simulink model "generator_model_2023"  (R2023a)
settings: Solver=ode15s  StartTime=0.0  StopTime=0.2  FixedStep=1e-6  MaxStep=1e-5  RelTol=1e-5  EnableMultiTasking=on
InitFcn:
  | Rs=0.42;
  | Ls=0.96e-3;
  | C_phi=92.1952e-3;
  | poles=8;
  | Rload=15;
model workspace (MAT data in the model file):
  D = Simulink.Parameter
  D.Value = 0
  D.DataType = 'double'
  D.Complexity = 'real'
  D.Dimensions = [1 1]
  Power_previous = Simulink.Parameter
  Power_previous.Value = 0
  Power_previous.DataType = 'auto'
  Power_previous.Complexity = 'real'
  Power_previous.Dimensions = [1 1]
  R_eq = Simulink.Parameter
  R_eq.Value = 100
  R_eq.DataType = 'double'
  R_eq.Complexity = 'real'
  R_eq.Dimensions = [1 1]
  direction = Simulink.Parameter
  direction.Value = 0
  direction.DataType = 'auto'
  direction.Complexity = 'real'
  direction.Dimensions = [1 1]
libraries: spsDiodeLib x6, spsSeriesRLCBranchLib x6, spsControlledVoltageSourceLib x3, ee_lib x2, spsVoltageMeasurementLib x2, spsCurrentMeasurementLib x1, spsGroundLib x1, spsParallelRLCBranchLib x1, sps_lib x1
settings Model: Creator=jwjansen  LastModifiedBy=maarten
settings SolverCC: AlgebraicLoopSolver=TrustRegion
settings DataIOCC: LimitDataPoints=on  SaveFormat=Array  ReturnWorkspaceOutputs=off
settings OptimizationCC: ExpressionDepthLimit=2147483647  LifeSpan=inf
settings DebuggingCC: UnderspecifiedInitializationDetection=Classic  MergeDetectMultiDrivingBlocksExec=none  SolverPrmCheckMsg=warning  FcnCallInpInsideContextMsg=warning  StateNameClashWarn=warning  SFUnexpectedBacktrackingDiag=warning  SFNoUnconditionalDefaultTransitionDiag=warning  SFExecutionAtInitializationDiag=none  ArithmeticOperatorsInVariantConditions=warning
settings HardwareCC: ProdBitPerPointer=32  ProdBitPerSizeT=32  ProdBitPerPtrDiffT=32  ProdLargestAtomicFloat=None  ProdIntDivRoundTo=Undefined  ProdEndianess=Unspecified  ProdWordSize=32  ProdHWDeviceType=32-bit Generic
settings ModelReferenceCC: EnableRefExpFcnMdlSchedulingChecks=on  PropagateSignalLabelsOutOfModel=off
settings SFSimCC: SimUseLocalCustomCode=off  SimParseCustomCode=off  CustomCodeUndefinedFunction=UseInterfaceOnly
settings RTWCC: RTWUseLocalCustomCode=off
settings CodeAppCC: StateflowObjectComments=on
settings GRTTargetCC: TargetLangStandard=C89/C90 (ANSI)  CombineOutputUpdateFcns=off  GRTInterface=on
settings ConfigComp: CovMetricSettings=dw  CovSaveCumulativeToWorkspaceVar=on  CovSaveSingleToWorkspaceVar=on  CovExternalEMLEnable=off
settings SimscapeCC: SimscapeNormalizeSystem=off

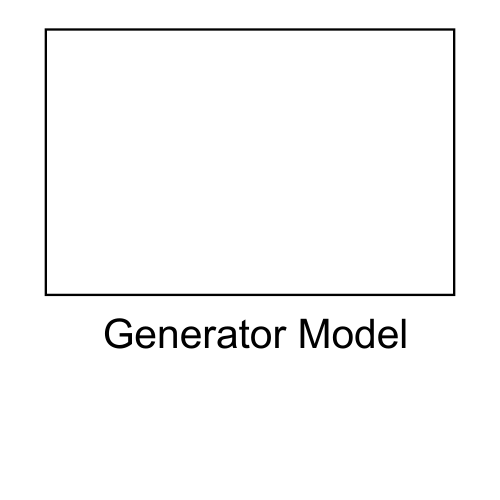
[thumbnail: Simulink's stored preview of the top-level diagram]
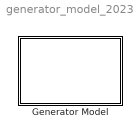
== system generator_model_2023 ==
  " Generator Model " : Subsystem

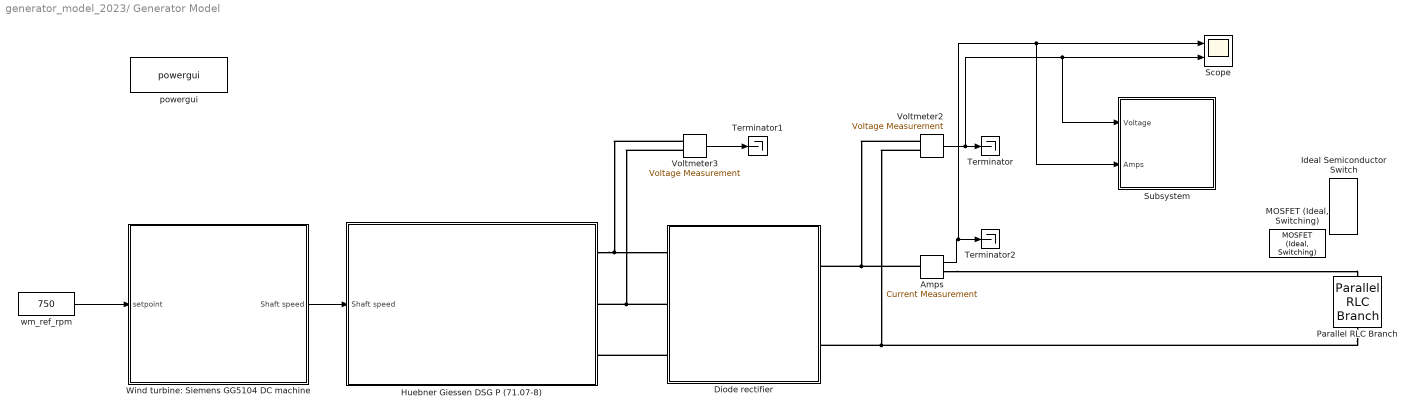
== system generator_model_2023/ Generator Model  ==
  Amps : spsCurrentMeasurementLib/Current Measurement  PhasorSimulation=off  OutputType=Complex  PSBequivalent=0
  Diode rectifier : Subsystem
  "Huebner Giessen DSG P (71.07-8) " : Subsystem
  Ideal Semiconductor Switch : ee_lib/Semiconductors & Converters/Ideal Semiconductor Switch  port_option=ee.enum.controlport.ps  Ron=0.001 Ohm  Goff=1e-6 1/Ohm  Vth=0.5 V  diode_param=ee.enum.converters.protectiondiode.none  diode_Vf=0.8 V  diode_Ron=0.001 Ohm  diode_Goff=1e-5 1/Ohm  diode_C=50e-9 F  diode_iRM=-235 A  diode_iF=300 A  diode_idot=-50 A/us  diode_trr_param=ee.enum.converters.diodetrr.trr_factor  diode_trr_factor=3  diode_trr=15 us  diode_Qrr=1500 s*uA
  "MOSFET (Ideal, Switching)" : ee_lib/Semiconductors & Converters/MOSFET (Ideal, Switching)  port_option=ee.enum.controlport.ps  Rds=0.01 Ohm  Goff=1e-6 1/Ohm  Vth=2 V  diode_param=ee.enum.converters.protectiondiode.none  diode_Vf=0.8 V  diode_Ron=0.001 Ohm  diode_Goff=1e-5 1/Ohm  diode_C=50e-9 F  diode_iRM=-235 A  diode_iF=300 A  diode_idot=-50 A/us  diode_trr_param=ee.enum.converters.diodeReverseParam.trr_factor  diode_trr_factor=3  diode_trr=15 us  diode_Qrr=1500 s*uA  ids_specify=off  ids_priority=None  ids=0 A  ids_nominal_specify=off  ids_nominal_unit=A  ids_nominal_value=1  vds_specify=off  vds_priority=None  vds=0 V  vds_nominal_specify=off  vds_nominal_unit=V  vds_nominal_value=1  vgs_specify=off  vgs_priority=None  vgs=0 V  vgs_nominal_specify=off  vgs_nominal_unit=V  vgs_nominal_value=1  thermal_loss_option=ee.enum.converters.thermalLossOption.constantvalues  Von_data=[0, 1.8, 3.2, 6, 10, 16; 0, 2, 5.5, 9.5, 15, 25] V  Tj=[298.15, 448.15] K  Iout_data=[0, 20, 40, 60, 80, 100] A  Eon_data=[0, 55.04, 124.57, 235.53, 362.12; 0, 71.25, 161.25, 304.88, 468.75] * 1e-6 J  Eoff_data=[0, 18, 30, 56.1, 76.5; 0, 22.5, 37.5, 70.13, 95.63] * 1e-6 J  Tj_loss=[298.15, 448.15] K  Iout_data_loss=[0, 10, 20, 30, 40] A  Eon_scalar=22.86e-3 J  Eoff_scalar=17.14e-3 J  Voff=300 V  Iout_scalar=600 A  diodeModelType=ee.enum.converters.diodeModelType.pwl  diodeTableType=ee.enum.diode.tableType.IfMat  diode_IfMat=[.07, .12, .19, 1.75, 4.24, 7.32, 11.2; .16, .3, .72, 2.14, 4.02, 6.35, 9.12] A  diode_VfMat=[.9, 1.15, 1.25, 1.5, 1.75, 2.17, 2.6, 2.85; .58, .68, .75, 1.1, 1.38, 1.77, 2.27, 2.7] V  diode_TjVec=[25, 125] degC  diode_VfVec=[.5, .7, .9, 1.3, 1.7, 2.1, 2.5] V  diode_IfVec=[.1, .2, .5, 1, 2, 4, 7, 10] A  diode_Vr=-600 V  diode_Ls=150 nH  diode_Erec=0.03 J  diode_rec_loss_model=ee.enum.diode.reverseRecoveryModel.fixed  diode_ErecVal=0 J  diode_ErecMat=zeros(2, 3) J  diode_TjrecVec=[298.15, 398.15] K  diode_IfrecVec=[.1, 1, 10] A  diode_VrecVal=10 V  diode_tFilter=1 / 1000 / 100 s  thermal_network_parameterization=ee.enum.thermalNetworkTopology.external  Rth=[.03, .2] K/W  Rth_Cauer=[.03, .1, .2] K/W  Rth_Foster=[.03, .2] K/W  thermal_mass_parameterization=ee.enum.thermalNetwork.timeconstant  thermal_mass=[3, 25] J/K  thermal_mass_Cauer=[3, 10, 25] J/K  thermal_mass_Foster=[33, 50] J/K  thermal_time_constant=[.1, 5] s  thermal_time_constant_Cauer=[.1, 1, 5] s  thermal_time_constant_Foster=[1, 10] s  thermal_mass_initial_temperatures=[25, 25] degC  thermal_mass_initial_temperatures_Cauer=[25, 25, 25] degC  junction_thermal_mass=0.1 J/K  Tvec_initial_Foster=[25, 25, 25, 25] degC  no_thermal_network=0  junction_temperature_specify=off  junction_temperature_priority=None  junction_temperature=25 degC  junction_temperature_nominal_specify=off  junction_temperature_nominal_unit=degC  junction_temperature_nominal_value=1  Qj_specify=off  Qj_priority=None  Qj=0 W  Qj_nominal_specify=off  Qj_nominal_unit=W  Qj_nominal_value=1
  Parallel RLC Branch : spsParallelRLCBranchLib/Parallel RLC Branch  LConnTagsString=a  RConnTagsString=__new0  BranchType=R  Resistance=R_eq  Inductance=1e-3  SetiL0=off  InitialCurrent=0  Capacitance=1e-6  Setx0=off  InitialVoltage=0  Measurements=Branch voltage and current
  Scope : Scope  NumInputPorts=2
  Subsystem : Subsystem
  Terminator : Terminator
  Terminator1 : Terminator
  Terminator2 : Terminator
  Voltmeter2 : spsVoltageMeasurementLib/Voltage Measurement  PhasorSimulation=off  OutputType=Complex  PSBequivalent=0
  Voltmeter3 : spsVoltageMeasurementLib/Voltage Measurement  PhasorSimulation=off  OutputType=Complex  PSBequivalent=0
  "Wind turbine: Siemens GG5104 DC machine " : Subsystem
  powergui : sps_lib/powergui  Priority=1  SimulationMode=Continuous  SampleTime=1e-6  frequency=60  Iterations=50  frequencyindice=0  Pbase=100e6  ErrMax=1e-4  UnitsV=kV  UnitsW=MW  buscounter=0  FunctionMessages=off  echomessages=off  EnableUseOfTLC=off  CurrentSourceSwitches=off  DisableSnubberDevices=off  DisableRonSwitches=off  DisableVfSwitches=off  DisplayEquations=off  AutomaticDiscreteSolvers=off  SolverType=Tustin  Interpol=off  ExternalGateDelay=off  methode=off  Ts=0  x0status=blocks  SPID=off  SwTol=0  HookPort=off  NonlinearTolerance=1e-4  nMaxIteration=100  ContinueOnMaxIteration=off  RestoreLinks=warning  ResistiveCurrentMeasurement=off  Frange=[0:2:500]  Ylog=off  Xlog=on  ShowGrid=off  save=off  variable=ZData  structure=0  ZoomFFT=off  StartTime=0.0  cycles=1  DisplayStyle=1  fundamental=60  FreqAxis=off  MaxFrequency=1000  frequencyindicesteady=1  RmsSteady=1  display=off
  wm_ref_rpm : Constant  Value=750
  wires:
  wm_ref_rpm/1 -> "Wind turbine: Siemens GG5104 DC machine "/1(setpoint)
  "Wind turbine: Siemens GG5104 DC machine "/1(Shaft speed) -> "Huebner Giessen DSG P (71.07-8) "/1(Shaft speed)
  Voltmeter2/1 -> Subsystem/1(Voltage), Scope/2, Terminator/1
  Voltmeter3/1 -> Terminator1/1
  Amps/1 -> Terminator2/1, Subsystem/2(Amps), Scope/1
  connections:
  "Huebner Giessen DSG P (71.07-8) "/RConn1 -- Voltmeter3/LConn1 -- Diode rectifier/LConn1
  Diode rectifier/LConn2 -- Voltmeter3/LConn2 -- "Huebner Giessen DSG P (71.07-8) "/RConn2
  Diode rectifier/LConn3 -- "Huebner Giessen DSG P (71.07-8) "/RConn3
  Voltmeter2/LConn1 -- Amps/LConn1 -- Diode rectifier/RConn1
  Voltmeter2/LConn2 -- Parallel RLC Branch/RConn1 -- Diode rectifier/RConn2
  Amps/RConn1 -- Parallel RLC Branch/LConn1

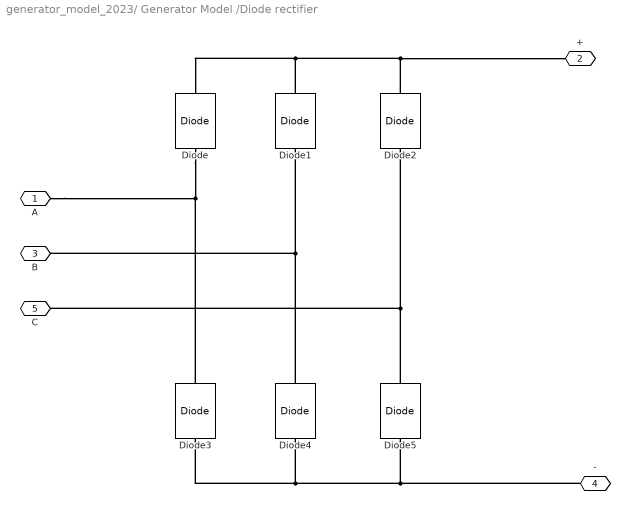
== system generator_model_2023/ Generator Model /Diode rectifier ==
  Diode{,1..5} (6 alike) : spsDiodeLib/Diode  Ron=0.01  Lon=0  Vf=0.85  IC=0  UseSnubber=off  Rs=500  Cs=250e-9  Measurements=off
  A : PMIOPort  Side=Left
  + : PMIOPort  Port=2  Side=Right
  B : PMIOPort  Port=3  Side=Left
  - : PMIOPort  Port=4  Side=Right
  C : PMIOPort  Port=5  Side=Left
  connections:
  Diode2/LConn1 -- C/RConn1 -- Diode5/RConn1
  +/RConn1 -- Diode2/RConn1 -- Diode1/RConn1 -- Diode/RConn1
  Diode3/LConn1 -- -/RConn1 -- Diode5/LConn1 -- Diode4/LConn1
  Diode3/RConn1 -- A/RConn1 -- Diode/LConn1
  Diode1/LConn1 -- B/RConn1 -- Diode4/RConn1

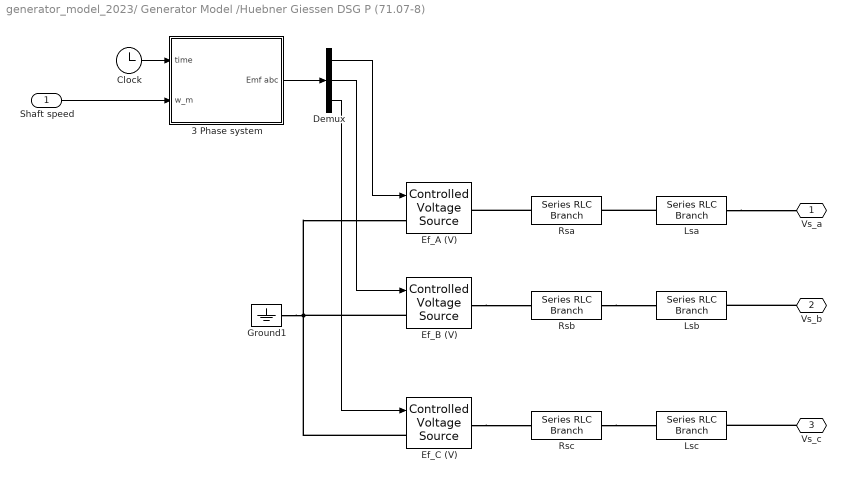
== system generator_model_2023/ Generator Model /Huebner Giessen DSG P (71.07-8)  ==
  Shaft speed : Inport
  "3 Phase system " : Subsystem
  Clock : Clock
  Demux : Demux  Outputs=3
  Ef_A (V) : spsControlledVoltageSourceLib/Controlled Voltage Source  Initialize=on  Source_Type=AC  Amplitude=0  Phase=0  Frequency=0  Measurements=None
  Ef_B (V) : spsControlledVoltageSourceLib/Controlled Voltage Source  Initialize=on  Source_Type=AC  Amplitude=0  Phase=0  Frequency=0  Measurements=None
  Ef_C (V) : spsControlledVoltageSourceLib/Controlled Voltage Source  Initialize=on  Source_Type=AC  Amplitude=0  Phase=0  Frequency=0  Measurements=None
  Ground1 : spsGroundLib/Ground  LConnTagsString=a
  Lsa : spsSeriesRLCBranchLib/Series RLC Branch  LConnTagsString=__new0  RConnTagsString=__new0  BranchType=L  Resistance=Rs  Inductance=Ls  SetiL0=off  InitialCurrent=0  Capacitance=1e-6  Setx0=off  InitialVoltage=0  Measurements=Branch current
  Lsb : spsSeriesRLCBranchLib/Series RLC Branch  LConnTagsString=__new0  RConnTagsString=__new0  BranchType=L  Resistance=Rs  Inductance=Ls  SetiL0=off  InitialCurrent=0  Capacitance=1e-6  Setx0=off  InitialVoltage=0  Measurements=Branch current
  Lsc : spsSeriesRLCBranchLib/Series RLC Branch  LConnTagsString=__new0  RConnTagsString=__new0  BranchType=L  Resistance=Rs  Inductance=Ls  SetiL0=on  InitialCurrent=0  Capacitance=1e-6  Setx0=off  InitialVoltage=0  Measurements=Branch current
  Rsa : spsSeriesRLCBranchLib/Series RLC Branch  LConnTagsString=__new0  RConnTagsString=__new0  BranchType=R  Resistance=Rs  Inductance=Ls  SetiL0=off  InitialCurrent=0  Capacitance=1e-6  Setx0=off  InitialVoltage=0  Measurements=Branch current
  Rsb : spsSeriesRLCBranchLib/Series RLC Branch  LConnTagsString=__new0  RConnTagsString=__new0  BranchType=R  Resistance=Rs  Inductance=Ls  SetiL0=off  InitialCurrent=0  Capacitance=1e-6  Setx0=off  InitialVoltage=0  Measurements=Branch current
  Rsc : spsSeriesRLCBranchLib/Series RLC Branch  LConnTagsString=__new0  RConnTagsString=__new0  BranchType=R  Resistance=Rs  Inductance=Ls  SetiL0=on  InitialCurrent=0  Capacitance=1e-6  Setx0=off  InitialVoltage=0  Measurements=Branch current
  Vs_a : PMIOPort  Side=Right
  Vs_b : PMIOPort  Port=2  Side=Right
  Vs_c : PMIOPort  Port=3  Side=Right
  wires:
  Demux/1 -> Ef_A (V)/1
  Demux/3 -> Ef_C (V)/1
  Demux/2 -> Ef_B (V)/1
  Shaft speed/1 -> "3 Phase system "/2(w_m)
  Clock/1 -> "3 Phase system "/1(time)
  "3 Phase system "/1("Emf abc ") -> Demux/1
  connections:
  Ef_B (V)/RConn1 -- Rsb/LConn1
  Lsa/RConn1 -- Vs_a/RConn1
  Vs_b/RConn1 -- Lsb/RConn1
  Ef_B (V)/LConn1 -- Ground1/LConn1 -- Ef_C (V)/LConn1 -- Ef_A (V)/LConn1
  Vs_c/RConn1 -- Lsc/RConn1
  Lsa/LConn1 -- Rsa/RConn1
  Ef_C (V)/RConn1 -- Rsc/LConn1
  Rsa/LConn1 -- Ef_A (V)/RConn1
  Rsb/RConn1 -- Lsb/LConn1
  Rsc/RConn1 -- Lsc/LConn1

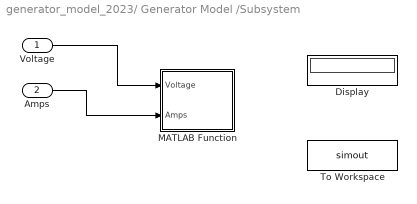
== system generator_model_2023/ Generator Model /Subsystem ==
  Voltage : Inport
  Amps : Inport  Port=2
  Display : Display
  MATLAB Function : MATLAB Function  TreatAsAtomicUnit=on  SystemSampleTime=0.1
  To Workspace : ToWorkspace  VariableName=simout  SaveFormat=Timeseries  SampleTime=-1
  wires:
  Voltage/1 -> MATLAB Function/1(Voltage)
  Amps/1 -> MATLAB Function/2(Amps)
  ? -> Display/1

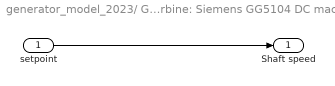
== system generator_model_2023/ Generator Model /Wind turbine: Siemens GG5104 DC machine  ==
  setpoint : Inport
  Shaft speed : Outport
  wires:
  setpoint/1 -> Shaft speed/1

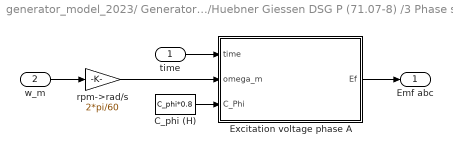
== system generator_model_2023/ Generator Model /Huebner Giessen DSG P (71.07-8) /3 Phase system  ==
  time : Inport
  w_m : Inport  Port=2
  C_phi (H) : Constant  Value=C_phi*0.8  VectorParams1D=off
  Excitation voltage phase A : Subsystem
  rpm->rad/s : Gain  Gain=2*pi/60
  "Emf abc " : Outport
  wires:
  w_m/1 -> rpm->rad/s/1
  C_phi (H)/1 -> Excitation voltage phase A/3(C_Phi)
  time/1 -> Excitation voltage phase A/1(time)
  rpm->rad/s/1 -> Excitation voltage phase A/2(omega_m)
  Excitation voltage phase A/1(Ef) -> "Emf abc "/1

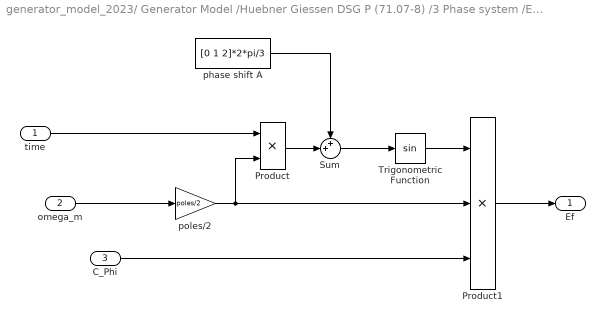
== system generator_model_2023/ Generator Model /Huebner Giessen DSG P (71.07-8) /3 Phase system /Excitation voltage phase A ==
  time : Inport
  omega_m : Inport  Port=2
  C_Phi : Inport  Port=3
  Product : Product  RndMeth=Zero
  Product1 : Product  Inputs=3  RndMeth=Zero
  Sum : Sum  Inputs=++|
  Trigonometric Function : Trigonometry
  phase shift A : Constant  Value=[0 1 2]*2*pi/3
  poles/2 : Gain  Gain=poles/2
  Ef : Outport
  wires:
  poles/2/1 -> Product/2, Product1/2
  Trigonometric Function/1 -> Product1/1
  phase shift A/1 -> Sum/1
  Product/1 -> Sum/2
  Product1/1 -> Ef/1
  C_Phi/1 -> Product1/3
  Sum/1 -> Trigonometric Function/1
  time/1 -> Product/1
  omega_m/1 -> poles/2/1

== matlab function generator_model_2023/ Generator Model /Subsystem/MATLAB Function ==
  settings: updateMethod=DISCRETE  sampleTime=0.1
  data: Voltage input; Amps input; direction parameter
function fcn(Voltage, Amps, direction)

Power = Voltage * Amps;

if Power < get_param('Power_previous','Value')
    %direction = direction;
end

set_param('Power_previous', 'Value', Power);
D = get_param('D', 'Value');
D = D + (0.1 * direction) - (0.1 * ~direction);
set_param('D', 'Value', D);

R_eq = Voltage;%D^2 * R;
set_param('R_eq', 'Value', R_eq);
